simulink model "tf2"  (R2024a)
settings: Solver=VariableStepAuto  StartTime=0.0  StopTime=10.0  RelTol=1e-3

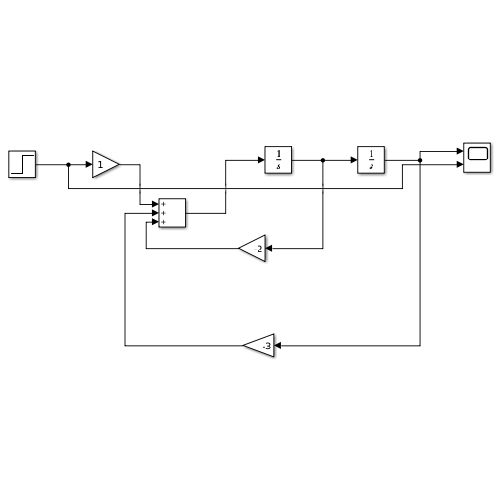
[thumbnail: Simulink's stored preview of the top-level diagram]
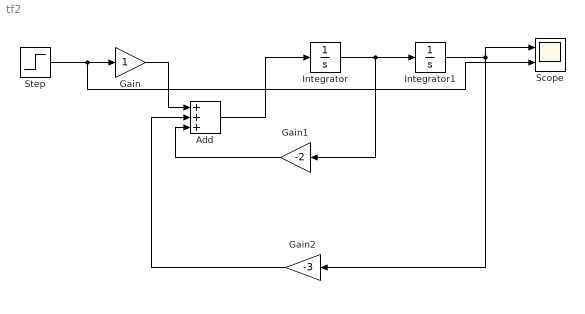
== system tf2 ==
  Add : Sum  Inputs=+++
  Gain : Gain
  Gain1 : Gain  Gain=-2
  Gain2 : Gain  Gain=-3
  Integrator : Integrator
  Integrator1 : Integrator  InitialCondition=0.5
  Scope : Scope  NumInputPorts=2
  Step : Step  SampleTime=0
  wires:
  Add/1 -> Integrator/1
  Integrator1/1 -> Gain2/1, Scope/1
  Gain/1 -> Add/1
  Gain2/1 -> Add/2
  Integrator/1 -> Gain1/1, Integrator1/1
  Step/1 -> Scope/2, Gain/1
  Gain1/1 -> Add/3
